simulink model "ProcessModel_copy"  (Simulink 7.9)
settings: Solver=VariableStepDiscrete  StartTime=0.0  StopTime=1000.0  RelTol=1e-3
settings Model: Creator=tsprock3  LastModifiedBy=tsprock3
settings DebuggingCC: SimStateOlderReleaseMsg=warning

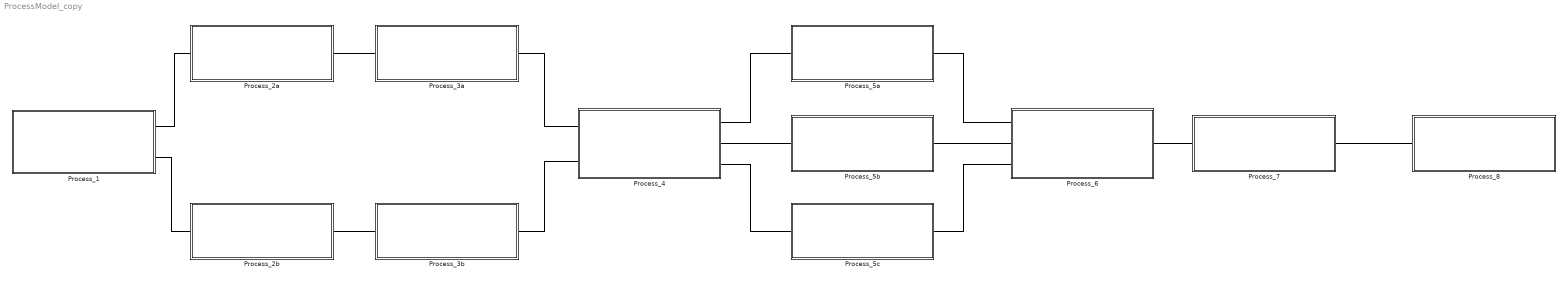
== system ProcessModel_copy ==
  Process_1 : Subsystem
  Process_2a : Subsystem
  Process_2b : Subsystem
  Process_3a : Subsystem
  Process_3b : Subsystem
  Process_4 : Subsystem
  Process_5a : Subsystem
  Process_5b : Subsystem
  Process_5c : Subsystem
  Process_6 : Subsystem
  Process_7 : Subsystem
  Process_8 : Subsystem
  connections:
  Process_1/RConn1 -- Process_2a/LConn1
  Process_2a/RConn1 -- Process_3a/LConn1
  Process_1/RConn2 -- Process_2b/LConn1
  Process_2b/RConn1 -- Process_3b/LConn1
  Process_3a/RConn1 -- Process_4/LConn1
  Process_3b/RConn1 -- Process_4/LConn2
  Process_4/RConn1 -- Process_5a/LConn1
  Process_4/RConn2 -- Process_5b/LConn1
  Process_4/RConn3 -- Process_5c/LConn1
  Process_5a/RConn1 -- Process_6/LConn1
  Process_5b/RConn1 -- Process_6/LConn2
  Process_5c/RConn1 -- Process_6/LConn3
  Process_6/RConn1 -- Process_7/LConn1
  Process_7/RConn1 -- Process_8/LConn1

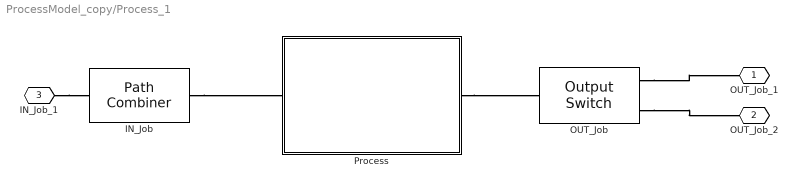
== system ProcessModel_copy/Process_1 ==
  IN_Job : PathCombiner  NumberInputPorts=1
  OUT_Job : OutputSwitch  NumberOutputPorts=2  SwitchingCriterion=Equiprobable  InitialSeed=4276
  Process : Subsystem
  OUT_Job_1 : PMIOPort  Port=1  Side=Right
  OUT_Job_2 : PMIOPort  Port=2  Side=Right
  IN_Job_1 : PMIOPort  Port=3  Side=Left
  connections:
  Process/RConn1 -- OUT_Job/LConn1
  IN_Job/RConn1 -- Process/LConn1
  OUT_Job/RConn1 -- OUT_Job_1/RConn1
  OUT_Job/RConn2 -- OUT_Job_2/RConn1
  IN_Job_1/RConn1 -- IN_Job/LConn1

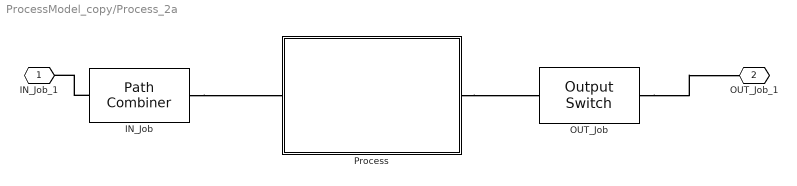
== system ProcessModel_copy/Process_2a ==
  IN_Job : PathCombiner  NumberInputPorts=1
  OUT_Job : OutputSwitch  NumberOutputPorts=1  SwitchingCriterion=Equiprobable  InitialSeed=7493
  Process : Subsystem
  IN_Job_1 : PMIOPort  Port=1  Side=Left
  OUT_Job_1 : PMIOPort  Port=2  Side=Right
  connections:
  Process/RConn1 -- OUT_Job/LConn1
  IN_Job/RConn1 -- Process/LConn1
  IN_Job/LConn1 -- IN_Job_1/RConn1
  OUT_Job/RConn1 -- OUT_Job_1/RConn1

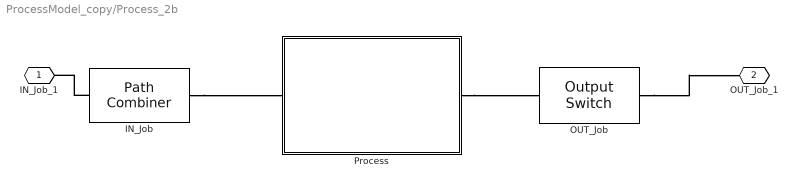
== system ProcessModel_copy/Process_2b ==
  IN_Job : PathCombiner  NumberInputPorts=1
  OUT_Job : OutputSwitch  NumberOutputPorts=1  SwitchingCriterion=Equiprobable  InitialSeed=10710
  Process : Subsystem
  IN_Job_1 : PMIOPort  Port=1  Side=Left
  OUT_Job_1 : PMIOPort  Port=2  Side=Right
  connections:
  Process/RConn1 -- OUT_Job/LConn1
  IN_Job/RConn1 -- Process/LConn1
  IN_Job/LConn1 -- IN_Job_1/RConn1
  OUT_Job/RConn1 -- OUT_Job_1/RConn1

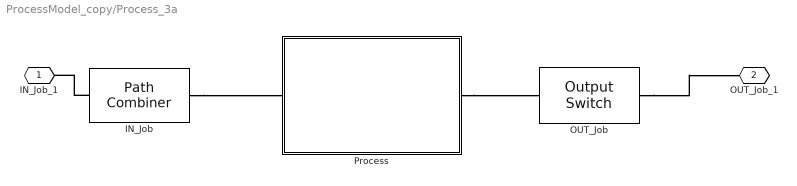
== system ProcessModel_copy/Process_3a ==
  IN_Job : PathCombiner  NumberInputPorts=1
  OUT_Job : OutputSwitch  NumberOutputPorts=1  SwitchingCriterion=Equiprobable  InitialSeed=13927
  Process : Subsystem
  IN_Job_1 : PMIOPort  Port=1  Side=Left
  OUT_Job_1 : PMIOPort  Port=2  Side=Right
  connections:
  Process/RConn1 -- OUT_Job/LConn1
  IN_Job/RConn1 -- Process/LConn1
  IN_Job/LConn1 -- IN_Job_1/RConn1
  OUT_Job/RConn1 -- OUT_Job_1/RConn1

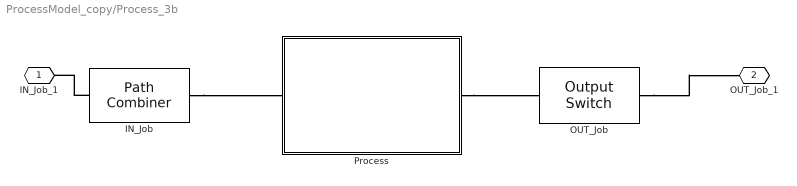
== system ProcessModel_copy/Process_3b ==
  IN_Job : PathCombiner  NumberInputPorts=1
  OUT_Job : OutputSwitch  NumberOutputPorts=1  SwitchingCriterion=Equiprobable  InitialSeed=17144
  Process : Subsystem
  IN_Job_1 : PMIOPort  Port=1  Side=Left
  OUT_Job_1 : PMIOPort  Port=2  Side=Right
  connections:
  Process/RConn1 -- OUT_Job/LConn1
  IN_Job/RConn1 -- Process/LConn1
  IN_Job/LConn1 -- IN_Job_1/RConn1
  OUT_Job/RConn1 -- OUT_Job_1/RConn1

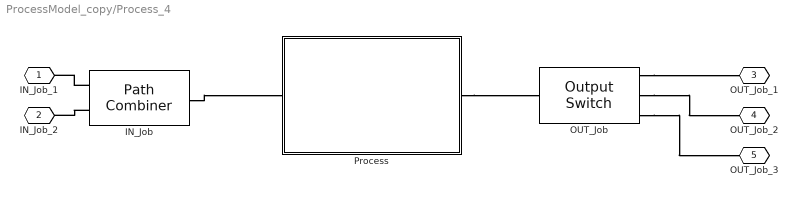
== system ProcessModel_copy/Process_4 ==
  IN_Job : PathCombiner  NumberInputPorts=2
  OUT_Job : OutputSwitch  SwitchingCriterion=Equiprobable  InitialSeed=20361
  Process : Subsystem
  IN_Job_1 : PMIOPort  Port=1  Side=Left
  IN_Job_2 : PMIOPort  Port=2  Side=Left
  OUT_Job_1 : PMIOPort  Port=3  Side=Right
  OUT_Job_2 : PMIOPort  Port=4  Side=Right
  OUT_Job_3 : PMIOPort  Port=5  Side=Right
  connections:
  Process/RConn1 -- OUT_Job/LConn1
  IN_Job/RConn1 -- Process/LConn1
  IN_Job/LConn1 -- IN_Job_1/RConn1
  IN_Job/LConn2 -- IN_Job_2/RConn1
  OUT_Job/RConn1 -- OUT_Job_1/RConn1
  OUT_Job/RConn2 -- OUT_Job_2/RConn1
  OUT_Job/RConn3 -- OUT_Job_3/RConn1

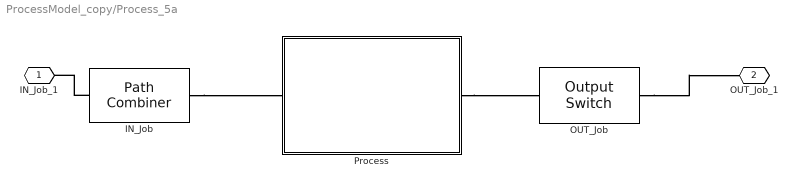
== system ProcessModel_copy/Process_5a ==
  IN_Job : PathCombiner  NumberInputPorts=1
  OUT_Job : OutputSwitch  NumberOutputPorts=1  SwitchingCriterion=Equiprobable  InitialSeed=23578
  Process : Subsystem
  IN_Job_1 : PMIOPort  Port=1  Side=Left
  OUT_Job_1 : PMIOPort  Port=2  Side=Right
  connections:
  Process/RConn1 -- OUT_Job/LConn1
  IN_Job/RConn1 -- Process/LConn1
  IN_Job/LConn1 -- IN_Job_1/RConn1
  OUT_Job/RConn1 -- OUT_Job_1/RConn1

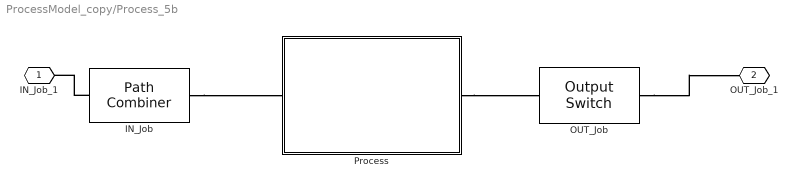
== system ProcessModel_copy/Process_5b ==
  IN_Job : PathCombiner  NumberInputPorts=1
  OUT_Job : OutputSwitch  NumberOutputPorts=1  SwitchingCriterion=Equiprobable  InitialSeed=26795
  Process : Subsystem
  IN_Job_1 : PMIOPort  Port=1  Side=Left
  OUT_Job_1 : PMIOPort  Port=2  Side=Right
  connections:
  Process/RConn1 -- OUT_Job/LConn1
  IN_Job/RConn1 -- Process/LConn1
  IN_Job/LConn1 -- IN_Job_1/RConn1
  OUT_Job/RConn1 -- OUT_Job_1/RConn1

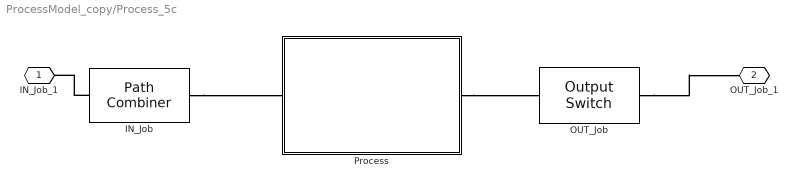
== system ProcessModel_copy/Process_5c ==
  IN_Job : PathCombiner  NumberInputPorts=1
  OUT_Job : OutputSwitch  NumberOutputPorts=1  SwitchingCriterion=Equiprobable  InitialSeed=30012
  Process : Subsystem
  IN_Job_1 : PMIOPort  Port=1  Side=Left
  OUT_Job_1 : PMIOPort  Port=2  Side=Right
  connections:
  Process/RConn1 -- OUT_Job/LConn1
  IN_Job/RConn1 -- Process/LConn1
  IN_Job/LConn1 -- IN_Job_1/RConn1
  OUT_Job/RConn1 -- OUT_Job_1/RConn1

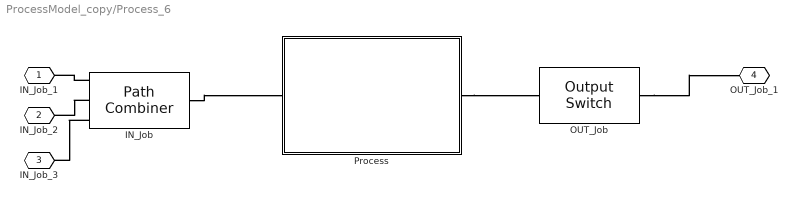
== system ProcessModel_copy/Process_6 ==
  IN_Job : PathCombiner
  OUT_Job : OutputSwitch  NumberOutputPorts=1  SwitchingCriterion=Equiprobable  InitialSeed=33229
  Process : Subsystem
  IN_Job_1 : PMIOPort  Port=1  Side=Left
  IN_Job_2 : PMIOPort  Port=2  Side=Left
  IN_Job_3 : PMIOPort  Port=3  Side=Left
  OUT_Job_1 : PMIOPort  Port=4  Side=Right
  connections:
  Process/RConn1 -- OUT_Job/LConn1
  IN_Job/RConn1 -- Process/LConn1
  IN_Job/LConn1 -- IN_Job_1/RConn1
  IN_Job/LConn2 -- IN_Job_2/RConn1
  IN_Job/LConn3 -- IN_Job_3/RConn1
  OUT_Job/RConn1 -- OUT_Job_1/RConn1

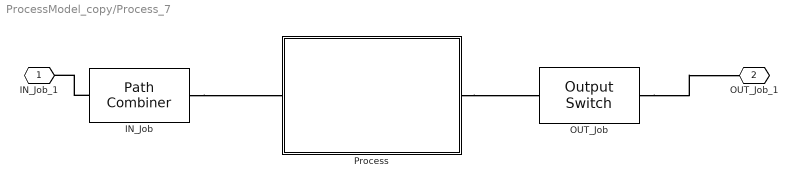
== system ProcessModel_copy/Process_7 ==
  IN_Job : PathCombiner  NumberInputPorts=1
  OUT_Job : OutputSwitch  NumberOutputPorts=1  SwitchingCriterion=Equiprobable  InitialSeed=36446
  Process : Subsystem
  IN_Job_1 : PMIOPort  Port=1  Side=Left
  OUT_Job_1 : PMIOPort  Port=2  Side=Right
  connections:
  Process/RConn1 -- OUT_Job/LConn1
  IN_Job/RConn1 -- Process/LConn1
  IN_Job/LConn1 -- IN_Job_1/RConn1
  OUT_Job/RConn1 -- OUT_Job_1/RConn1

== system ProcessModel_copy/Process_8 ==
  IN_Job : PathCombiner  NumberInputPorts=1
  OUT_Job : OutputSwitch  NumberOutputPorts=1  SwitchingCriterion=Equiprobable  InitialSeed=39663
  Process : Subsystem
  IN_Job_1 : PMIOPort  Port=1  Side=Left
  OUT_Job_1 : PMIOPort  Port=2  Side=Right
  connections:
  Process/RConn1 -- OUT_Job/LConn1
  IN_Job/RConn1 -- Process/LConn1
  IN_Job/LConn1 -- IN_Job_1/RConn1
  OUT_Job/RConn1 -- OUT_Job_1/RConn1

== system ProcessModel_copy/Process_1/Process ==
  Event-Based Random Number : EventBasedRandomNumber  Distribution=Gaussian (normal)  minUnif=1  meanNorm=5  Seed=31208
  FIFO Queue : FIFOQueue  Capacity=inf
  N-Server : NServer  NumberOfServers=inf  ServiceTimeFrom=Signal port t
  Job_OUT : PMIOPort  Port=1  Side=Right
  Job_IN : PMIOPort  Port=2  Side=Left
  wires:
  Event-Based Random Number/1 -> N-Server/1
  connections:
  Job_IN/RConn1 -- FIFO Queue/LConn1
  Job_OUT/RConn1 -- N-Server/RConn1
  FIFO Queue/RConn1 -- N-Server/LConn1

== system ProcessModel_copy/Process_2a/Process ==
  Event-Based Random Number : EventBasedRandomNumber  Distribution=Gaussian (normal)  minUnif=1  meanNorm=5  Seed=34425
  FIFO Queue : FIFOQueue  Capacity=inf
  N-Server : NServer  NumberOfServers=inf  ServiceTimeFrom=Signal port t
  Job_OUT : PMIOPort  Port=1  Side=Right
  Job_IN : PMIOPort  Port=2  Side=Left
  wires:
  Event-Based Random Number/1 -> N-Server/1
  connections:
  Job_IN/RConn1 -- FIFO Queue/LConn1
  Job_OUT/RConn1 -- N-Server/RConn1
  FIFO Queue/RConn1 -- N-Server/LConn1

== system ProcessModel_copy/Process_2b/Process ==
  Event-Based Random Number : EventBasedRandomNumber  Distribution=Gaussian (normal)  minUnif=1  meanNorm=5  Seed=37642
  FIFO Queue : FIFOQueue  Capacity=inf
  N-Server : NServer  NumberOfServers=inf  ServiceTimeFrom=Signal port t
  Job_OUT : PMIOPort  Port=1  Side=Right
  Job_IN : PMIOPort  Port=2  Side=Left
  wires:
  Event-Based Random Number/1 -> N-Server/1
  connections:
  Job_IN/RConn1 -- FIFO Queue/LConn1
  Job_OUT/RConn1 -- N-Server/RConn1
  FIFO Queue/RConn1 -- N-Server/LConn1

== system ProcessModel_copy/Process_3a/Process ==
  Event-Based Random Number : EventBasedRandomNumber  Distribution=Gaussian (normal)  minUnif=1  meanNorm=5  Seed=40859
  FIFO Queue : FIFOQueue  Capacity=inf
  N-Server : NServer  NumberOfServers=inf  ServiceTimeFrom=Signal port t
  Job_OUT : PMIOPort  Port=1  Side=Right
  Job_IN : PMIOPort  Port=2  Side=Left
  wires:
  Event-Based Random Number/1 -> N-Server/1
  connections:
  Job_IN/RConn1 -- FIFO Queue/LConn1
  Job_OUT/RConn1 -- N-Server/RConn1
  FIFO Queue/RConn1 -- N-Server/LConn1

== system ProcessModel_copy/Process_3b/Process ==
  Event-Based Random Number : EventBasedRandomNumber  Distribution=Gaussian (normal)  minUnif=1  meanNorm=5  Seed=44076
  FIFO Queue : FIFOQueue  Capacity=inf
  N-Server : NServer  NumberOfServers=inf  ServiceTimeFrom=Signal port t
  Job_OUT : PMIOPort  Port=1  Side=Right
  Job_IN : PMIOPort  Port=2  Side=Left
  wires:
  Event-Based Random Number/1 -> N-Server/1
  connections:
  Job_IN/RConn1 -- FIFO Queue/LConn1
  Job_OUT/RConn1 -- N-Server/RConn1
  FIFO Queue/RConn1 -- N-Server/LConn1

== system ProcessModel_copy/Process_4/Process ==
  Event-Based Random Number : EventBasedRandomNumber  Distribution=Gaussian (normal)  minUnif=1  meanNorm=5  Seed=47293
  FIFO Queue : FIFOQueue  Capacity=inf
  N-Server : NServer  NumberOfServers=inf  ServiceTimeFrom=Signal port t
  Job_OUT : PMIOPort  Port=1  Side=Right
  Job_IN : PMIOPort  Port=2  Side=Left
  wires:
  Event-Based Random Number/1 -> N-Server/1
  connections:
  Job_IN/RConn1 -- FIFO Queue/LConn1
  Job_OUT/RConn1 -- N-Server/RConn1
  FIFO Queue/RConn1 -- N-Server/LConn1

== system ProcessModel_copy/Process_5a/Process ==
  Event-Based Random Number : EventBasedRandomNumber  Distribution=Gaussian (normal)  minUnif=1  meanNorm=5  Seed=50510
  FIFO Queue : FIFOQueue  Capacity=inf
  N-Server : NServer  NumberOfServers=inf  ServiceTimeFrom=Signal port t
  Job_OUT : PMIOPort  Port=1  Side=Right
  Job_IN : PMIOPort  Port=2  Side=Left
  wires:
  Event-Based Random Number/1 -> N-Server/1
  connections:
  Job_IN/RConn1 -- FIFO Queue/LConn1
  Job_OUT/RConn1 -- N-Server/RConn1
  FIFO Queue/RConn1 -- N-Server/LConn1

== system ProcessModel_copy/Process_5b/Process ==
  Event-Based Random Number : EventBasedRandomNumber  Distribution=Gaussian (normal)  minUnif=1  meanNorm=5  Seed=53727
  FIFO Queue : FIFOQueue  Capacity=inf
  N-Server : NServer  NumberOfServers=inf  ServiceTimeFrom=Signal port t
  Job_OUT : PMIOPort  Port=1  Side=Right
  Job_IN : PMIOPort  Port=2  Side=Left
  wires:
  Event-Based Random Number/1 -> N-Server/1
  connections:
  Job_IN/RConn1 -- FIFO Queue/LConn1
  Job_OUT/RConn1 -- N-Server/RConn1
  FIFO Queue/RConn1 -- N-Server/LConn1

== system ProcessModel_copy/Process_5c/Process ==
  Event-Based Random Number : EventBasedRandomNumber  Distribution=Gaussian (normal)  minUnif=1  meanNorm=5  Seed=56944
  FIFO Queue : FIFOQueue  Capacity=inf
  N-Server : NServer  NumberOfServers=inf  ServiceTimeFrom=Signal port t
  Job_OUT : PMIOPort  Port=1  Side=Right
  Job_IN : PMIOPort  Port=2  Side=Left
  wires:
  Event-Based Random Number/1 -> N-Server/1
  connections:
  Job_IN/RConn1 -- FIFO Queue/LConn1
  Job_OUT/RConn1 -- N-Server/RConn1
  FIFO Queue/RConn1 -- N-Server/LConn1

== system ProcessModel_copy/Process_6/Process ==
  Event-Based Random Number : EventBasedRandomNumber  Distribution=Gaussian (normal)  minUnif=1  meanNorm=5  Seed=60161
  FIFO Queue : FIFOQueue  Capacity=inf
  N-Server : NServer  NumberOfServers=inf  ServiceTimeFrom=Signal port t
  Job_OUT : PMIOPort  Port=1  Side=Right
  Job_IN : PMIOPort  Port=2  Side=Left
  wires:
  Event-Based Random Number/1 -> N-Server/1
  connections:
  Job_IN/RConn1 -- FIFO Queue/LConn1
  Job_OUT/RConn1 -- N-Server/RConn1
  FIFO Queue/RConn1 -- N-Server/LConn1

== system ProcessModel_copy/Process_7/Process ==
  Event-Based Random Number : EventBasedRandomNumber  Distribution=Gaussian (normal)  minUnif=1  meanNorm=5  Seed=63378
  FIFO Queue : FIFOQueue  Capacity=inf
  N-Server : NServer  NumberOfServers=inf  ServiceTimeFrom=Signal port t
  Job_OUT : PMIOPort  Port=1  Side=Right
  Job_IN : PMIOPort  Port=2  Side=Left
  wires:
  Event-Based Random Number/1 -> N-Server/1
  connections:
  Job_IN/RConn1 -- FIFO Queue/LConn1
  Job_OUT/RConn1 -- N-Server/RConn1
  FIFO Queue/RConn1 -- N-Server/LConn1

== system ProcessModel_copy/Process_8/Process ==
  Event-Based Random Number : EventBasedRandomNumber  Distribution=Gaussian (normal)  minUnif=1  meanNorm=5  Seed=1059
  FIFO Queue : FIFOQueue  Capacity=inf
  N-Server : NServer  NumberOfServers=inf  ServiceTimeFrom=Signal port t
  Job_OUT : PMIOPort  Port=1  Side=Right
  Job_IN : PMIOPort  Port=2  Side=Left
  wires:
  Event-Based Random Number/1 -> N-Server/1
  connections:
  Job_IN/RConn1 -- FIFO Queue/LConn1
  Job_OUT/RConn1 -- N-Server/RConn1
  FIFO Queue/RConn1 -- N-Server/LConn1
